simulink model "latest_exp"  (R2020a)
settings: Solver=ode1  StartTime=0.0  StopTime=20  FixedStep=0.001  RelTol=1e-3  EnableMultiTasking=on
PostLoadFcn:
  | qc_set_target_type(getConfigSet(bdroot, 'QUARC Default Target Configuration'));
model workspace (MAT data in the model file):
  b0 = 2500
values from neighbouring files (symbols this model uses):
  A = [0 0 1 0 ... (first row only)    [lqrintctrl.m]
  B = [0;0;51.5346;-49.3846]    [lqrintctrl.m]
  C = [1 0 0 0;0 1 0 0]    [lqrintctrl.m]
  D = [0;0]    [lqrintctrl.m]
libraries: simulink_extras x6, simulink x2
settings Model: ExtModeTrigDuration=10000  ExtModeTrigDurationFloating=10000  Creator=Rchan  LastModifiedBy=frank
settings SolverCC: PositivePriorityOrder=on
settings DataIOCC: LimitDataPoints=on  SaveFormat=Array  ReturnWorkspaceOutputs=off
settings OptimizationCC: ExpressionDepthLimit=2147483647  InitFltsAndDblsToZero=on  LifeSpan=inf
settings DebuggingCC: SaveWithParameterizedLinksMsg=none  UnderspecifiedInitializationDetection=Classic  MergeDetectMultiDrivingBlocksExec=none  SolverPrmCheckMsg=warning  MultiTaskDSMMsg=warning  MultiTaskCondExecSysMsg=none  FcnCallInpInsideContextMsg=warning  StateNameClashWarn=warning  SFUnexpectedBacktrackingDiag=warning  SFNoUnconditionalDefaultTransitionDiag=warning  SFExecutionAtInitializationDiag=none  ArithmeticOperatorsInVariantConditions=warning
settings HardwareCC: ProdBitPerPointer=32  ProdBitPerSizeT=32  ProdBitPerPtrDiffT=32  ProdLargestAtomicFloat=None  ProdIntDivRoundTo=Undefined  ProdEndianess=Unspecified  ProdWordSize=32  ProdHWDeviceType=32-bit Generic
settings ModelReferenceCC: PropagateSignalLabelsOutOfModel=off
settings SFSimCC: SimUseLocalCustomCode=off  CustomCodeUndefinedFunction=UseInterfaceOnly
settings RTWCC: Description=QUARC Win64 Target  SystemTargetFile=quarc_win64.tlc  TemplateMakefile=quarc_default_tmf  RTWUseLocalCustomCode=off
settings CodeAppCC: StateflowObjectComments=on
settings STFCustomTargetCC: TargetPreCompLibLocation=C:\PROGRA~3\QUARC\lib\2017a\win64\release  ConcurrentExecutionCompliant=on  CPPClassGenCompliant=on  GRTInterface=on  SystemTargetFile=quarc_win64.tlc
settings GRTTargetCC: TargetPreCompLibLocation=C:\PROGRA~3\QUARC\lib\2017a\win64\release  TargetLangStandard=C89/C90 (ANSI)  ParMdlRefBuildCompliant=off  CompOptLevelCompliant=off  CombineOutputUpdateFcns=off  MatFileLogging=off  GRTInterface=on  UseToolchainInfoCompliant=off  ExtMode=on  ExtModeMexFile=quarc_comm
settings ConfigComp: CovMetricSettings=dw  CovHtmlReporting=on  CovSaveCumulativeToWorkspaceVar=on  CovSaveSingleToWorkspaceVar=on  CovExternalEMLEnable=off

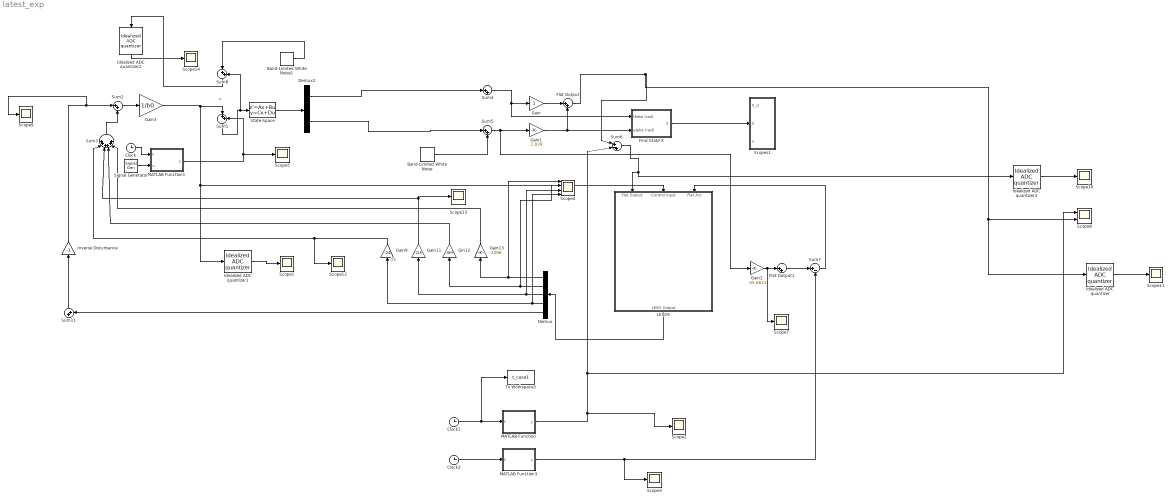
== system latest_exp ==
  note: -35
  note: u
  Band-Limited White Noise : simulink/Sources/Band-Limited White Noise  Cov=[1e-14]  Ts=0.001  seed=[2371]
  Band-Limited White Noise1 : simulink/Sources/Band-Limited White Noise  Cov=[1e-13]  Ts=0.001  seed=[2330]
  Clock : Clock
  Clock1 : Clock
  Clock2 : Clock
  Demux : Demux  Outputs=5
  Demux2 : Demux  Outputs=2
  Find State X : Subsystem
  Flat Output : Sum  Inputs=|++
  Flat Output1 : Sum  Inputs=|++
  Gain : Gain
  Gain1 : Gain  Gain=1.039
  Gain11 : Gain  Gain=-216
  Gain13 : Gain  Gain=-1296
  Gain2 : Gain  Gain=-45.6621
  Gain3 : Gain  Gain=1/b0
  Gain9 : Gain  Gain=-24
  Gin12 : Gain  Gain=-864
  Idealized ADC quantizer : simulink_extras/Additional Discrete/Idealized ADC quantizer  NumberOfConverterBits=12  Vmin=0  Vmax=5  OutputDataType=int16  OutputNegativeValues=off
  Idealized ADC quantizer1 : simulink_extras/Additional Discrete/Idealized ADC quantizer  NumberOfConverterBits=12  Vmin=-2  Vmax=2  OutputDataType=int16  OutputNegativeValues=on
  Idealized ADC quantizer2 : simulink_extras/Additional Discrete/Idealized ADC quantizer  NumberOfConverterBits=12  Vmin=-5  Vmax=5  OutputDataType=int16  OutputNegativeValues=on
  Idealized ADC quantizer3 : simulink_extras/Additional Discrete/Idealized ADC quantizer  NumberOfConverterBits=16  Vmin=-5  Vmax=5  OutputDataType=int16  OutputNegativeValues=on
  Inverse Disturbance : Gain  Gain=-1
  LESO5 : Subsystem
  MATLAB Function : MATLAB Function  TreatAsAtomicUnit=on
  MATLAB Function1 : MATLAB Function  TreatAsAtomicUnit=on
  MATLAB Function3 : MATLAB Function  TreatAsAtomicUnit=on
  Scope{1..3,5,7,9..14} (11 alike) : Scope
  Scope4 : Scope  NumInputPorts=4
  Scope8 : Scope  NumInputPorts=2
  Scopes1 : Subsystem
  Signal Generator : SignalGenerator  WaveForm=square  Amplitude=0.05  Frequency=0.5  Units=rad/sec
  State-Space : StateSpace  A=A  B=B  C=C  D=D  InitialCondition=[0,0,0,0]
  Sum{1..2,4..5,8,11} (6 alike) : Sum  Inputs=|++
  Sum3 : Sum  Inputs=++++++
  Sum6 : Sum  Inputs=|+-+
  Sum7 : Sum  Inputs=|+-
  To Workspace3 : ToWorkspace  VariableName=t_case1  SampleTime=-1
  wires:
  MATLAB Function3/1(y) -> Scope3/1, Sum7/2
  Clock2/1 -> MATLAB Function3/1(t)
  Gain13/1 -> Sum3/5
  Demux/3 -> Scope4/3, Gain11/1
  Sum2/1 -> Gain3/1
  Demux/5 -> Sum11/2
  Find State X/1(X) -> Scopes1/2(X)
  Demux/4 -> Gain9/1, Scope4/4
  Gain2/1 -> Scope7/1, Flat Output1/1
  Sum3/1 -> Sum2/2
  Sum11/1 -> Inverse Disturbance/1
  Gain9/1 -> Scope12/1, Sum3/2
  Gain3/1 -> Sum1/1, Idealized ADC quantizer1/1, LESO5/2(Control Input)
  Sum6/1 -> Idealized ADC quantizer3/1, LESO5/1(Flat Output)
  Flat Output1/1 -> Sum7/1
  MATLAB Function/1(y) -> Scope2/1, Sum6/2, Scope8/1
  Inverse Disturbance/1 -> Scope9/1, Sum2/1
  Sum4/1 -> Find State X/1(theta (rad)), Gain/1
  Sum7/1 -> LESO5/3("Flat Acc ")
  Gain11/1 -> Scope13/1, Sum3/3
  Demux/2 -> Scope4/2, Gin12/1
  Demux/1 -> Scope4/1, Gain13/1
  Demux2/1 -> Sum4/1
  Demux2/2 -> Sum5/1
  Gin12/1 -> Sum3/4
  LESO5/1(LESO Output) -> Demux/1
  Gain1/1 -> Find State X/2(alpha (rad)), Flat Output/2
  Gain/1 -> Flat Output/1
  Sum5/1 -> Gain2/1, Gain1/1
  Clock1/1 -> To Workspace3/1, MATLAB Function/1(t)
  State-Space/1 -> Demux2/1
  Idealized ADC quantizer/1 -> Scope11/1
  Idealized ADC quantizer1/1 -> Scope1/1
  Signal Generator/1 -> MATLAB Function1/2(u)
  MATLAB Function1/1(y) -> Scope5/1, Sum1/2
  Sum1/1 -> Sum8/2, State-Space/1
  Clock/1 -> MATLAB Function1/1(t)
  Band-Limited White Noise1/1 -> Sum8/1
  Flat Output/1 -> Idealized ADC quantizer/1, Scope8/2, Sum6/1
  Band-Limited White Noise/1 -> Sum5/2
  Sum8/1 -> Idealized ADC quantizer2/1
  Idealized ADC quantizer2/1 -> Scope14/1
  Idealized ADC quantizer3/1 -> Scope10/1

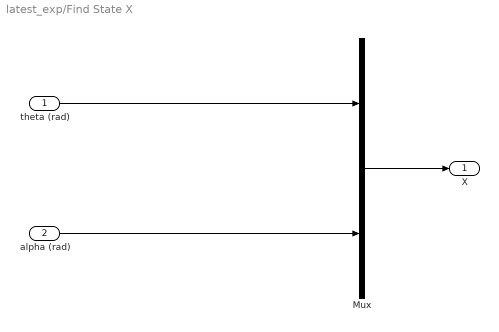
== system latest_exp/Find State X ==
  theta (rad) : Inport
  alpha (rad) : Inport  Port=2
  Mux : Mux  Inputs=2
  X : Outport
  wires:
  alpha (rad)/1 -> Mux/2
  Mux/1 -> X/1
  theta (rad)/1 -> Mux/1

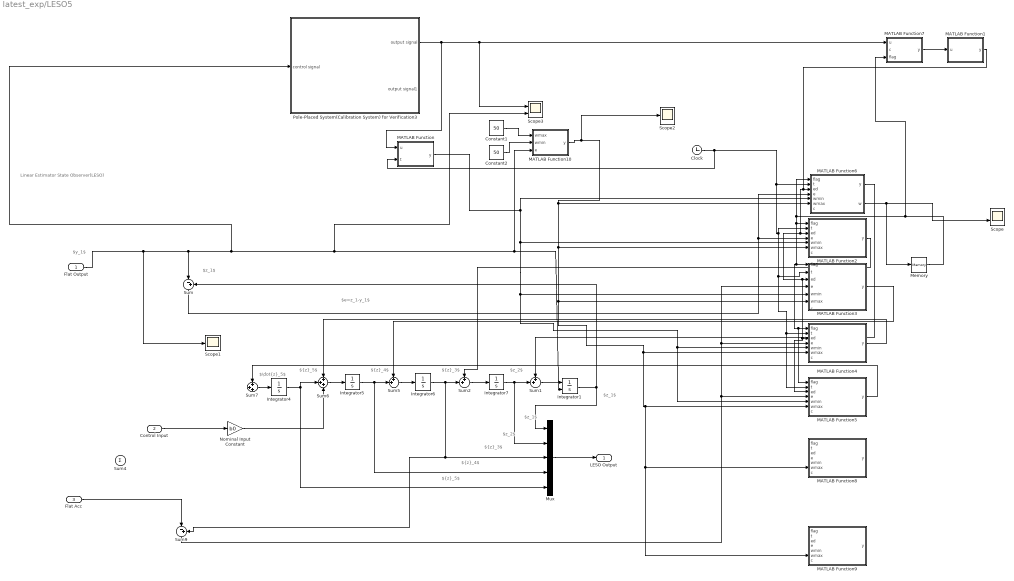
== system latest_exp/LESO5 ==
  note: $e=z_1-y_1$
  note: ${z}_5$
  note: $\dot{z}_5$
  note: ${z}_4$
  note: ${z}_3$
  note: $z_2$
  note: $z_1$
  note: $y_1$
  note: $z_1$
  note: Linear Estimator State Observer(LESO)
  note: $z_1$
  note: $z_2$
  note: ${z}_3$
  note: ${z}_4$
  note: ${z}_5$
  Flat Output : Inport
  Control Input : Inport  Port=2
  "Flat Acc " : Inport  Port=3
  Clock : Clock
  Constant1 : Constant  Value=50
  Constant2 : Constant  Value=50
  Integrator1 : Integrator  InitialConditionSource=external
  Integrator{4..7} (4 alike) : Integrator
  MATLAB Function : MATLAB Function  TreatAsAtomicUnit=on
  MATLAB Function1 : MATLAB Function  TreatAsAtomicUnit=on
  MATLAB Function10 : MATLAB Function  TreatAsAtomicUnit=on
  MATLAB Function2 : MATLAB Function  TreatAsAtomicUnit=on
  MATLAB Function3 : MATLAB Function  TreatAsAtomicUnit=on
  MATLAB Function4 : MATLAB Function  TreatAsAtomicUnit=on
  MATLAB Function5 : MATLAB Function  TreatAsAtomicUnit=on
  MATLAB Function6 : MATLAB Function  TreatAsAtomicUnit=on
  MATLAB Function7 : MATLAB Function  TreatAsAtomicUnit=on
  MATLAB Function8 : MATLAB Function  TreatAsAtomicUnit=on
  MATLAB Function9 : MATLAB Function  TreatAsAtomicUnit=on
  Memory : Memory
  Mux : Mux  Inputs=5
  Nominal Input Constant : Gain  Gain=b0
  Pole-Placed System(Calibration System) for Verification3 : Subsystem
  Scope : Scope  NumInputPorts=2
  Scope1 : Scope
  Scope2 : Scope
  Scope3 : Scope  NumInputPorts=2
  Sum : Sum  Inputs=|-+
  Sum1 : Sum  Inputs=++|
  Sum2 : Sum  Inputs=++|
  Sum4 : Sum  Inputs=+|
  Sum5 : Sum  Inputs=++|
  Sum6 : Sum  Inputs=+++
  Sum7 : Sum  Inputs=+++
  Sum9 : Sum  Inputs=|-+
  LESO Output : Outport
  wires:
  Integrator7/1 -> Mux/2, Sum1/2
  Integrator6/1 -> Sum9/2, Mux/3, Sum2/2
  Sum1/1 -> Integrator1/1
  Integrator4/1 -> Mux/5, Sum6/2
  Nominal Input Constant/1 -> Sum6/3
  Mux/1 -> LESO Output/1
  Sum2/1 -> Integrator7/1
  Sum5/1 -> Integrator6/1
  Integrator1/1 -> Sum/2, Mux/1
  Control Input/1 -> Nominal Input Constant/1
  Sum6/1 -> Integrator5/1
  Sum7/1 -> Integrator4/1
  Integrator5/1 -> Mux/4, Sum5/2
  MATLAB Function10/1(y) -> Scope2/1, MATLAB Function9/6(wmax), MATLAB Function8/6(wmax), MATLAB Function5/6(wmax), MATLAB Function4/6(wmax), MATLAB Function3/6(wmax), MATLAB Function2/6(wmax), MATLAB Function6/6(wmax)
  MATLAB Function/1(y) -> MATLAB Function5/5(wmin), MATLAB Function4/5(wmin), MATLAB Function3/5(wmin), MATLAB Function2/5(wmin), MATLAB Function6/5(wmin)
  ? -> MATLAB Function7/2(c), MATLAB Function5/7(c), MATLAB Function4/7(c), MATLAB Function3/7(c), MATLAB Function2/7(c), MATLAB Function6/7(c)
  MATLAB Function6/1(y) -> Sum1/1
  MATLAB Function2/1(y) -> Sum2/1
  MATLAB Function4/1(y) -> Sum6/1
  MATLAB Function5/1(y) -> Sum7/1
  Clock/1 -> MATLAB Function/2(t), MATLAB Function4/2(t), MATLAB Function5/2(t), MATLAB Function3/2(t), MATLAB Function2/2(t), MATLAB Function6/2(t)
  MATLAB Function6/2(w) -> Memory/1, Scope/2
  Flat Output/1 -> Scope1/1, Pole-Placed System(Calibration System) for Verification3/1(control signal), MATLAB Function10/3(e), Integrator1/2, Scope3/2, Sum/1
  Pole-Placed System(Calibration System) for Verification3/1(output signal) -> MATLAB Function/1(u), Scope3/1, MATLAB Function7/1(u)
  Memory/1 -> MATLAB Function7/3(flag), MATLAB Function2/1(flag), MATLAB Function3/1(flag), MATLAB Function4/1(flag), MATLAB Function5/1(flag), MATLAB Function6/1(flag)
  MATLAB Function7/1(y) -> MATLAB Function1/1(u)
  MATLAB Function1/1(y) -> MATLAB Function5/3(ed), MATLAB Function4/3(ed), MATLAB Function3/3(ed), MATLAB Function2/3(ed), MATLAB Function6/3(ed)
  Sum/1 -> MATLAB Function2/4(e), MATLAB Function6/4(e)
  MATLAB Function3/1(y) -> Sum5/1
  "Flat Acc "/1 -> Sum9/1
  Sum9/1 -> MATLAB Function3/4(e), MATLAB Function4/4(e), MATLAB Function5/4(e)
  Constant1/1 -> MATLAB Function10/1(wmax)
  Constant2/1 -> MATLAB Function10/2(wmin)

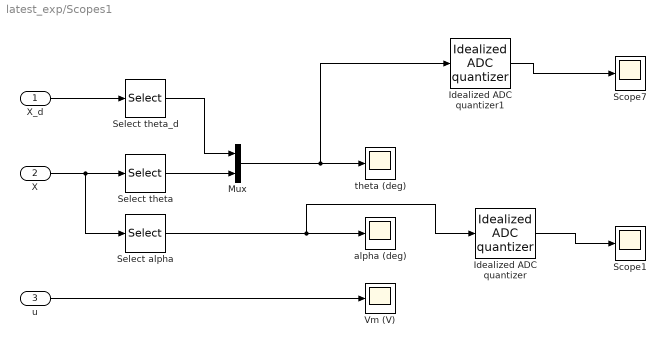
== system latest_exp/Scopes1 ==
  X_d : Inport
  X : Inport  Port=2
  u : Inport  Port=3
  Idealized ADC quantizer : simulink_extras/Additional Discrete/Idealized ADC quantizer  NumberOfConverterBits=12  Vmin=-2  Vmax=2  OutputDataType=int16  OutputNegativeValues=on
  Idealized ADC quantizer1 : simulink_extras/Additional Discrete/Idealized ADC quantizer  NumberOfConverterBits=12  Vmin=0  Vmax=5  OutputDataType=single  OutputNegativeValues=off
  Mux : Mux  Inputs=2
  Scope1 : Scope
  Scope7 : Scope
  Select alpha : Selector  InputPortWidth=2  IndexOptions=Index vector (dialog)  Indices=2  OutputSizes=[(-2)]
  Select theta : Selector  InputPortWidth=2  IndexOptions=Index vector (dialog)  Indices=1  OutputSizes=[(-2)]
  Select theta_d : Selector  InputPortWidth=4  IndexOptions=Index vector (dialog)  Indices=1  OutputSizes=[(-2)]
  Vm (V) : Scope
  alpha (deg) : Scope
  theta (deg) : Scope
  wires:
  u/1 -> Vm (V)/1
  X_d/1 -> Select theta_d/1
  X/1 -> Select alpha/1, Select theta/1
  Select theta_d/1 -> Mux/1
  Select theta/1 -> Mux/2
  Select alpha/1 -> Idealized ADC quantizer/1, alpha (deg)/1
  Mux/1 -> Idealized ADC quantizer1/1, theta (deg)/1
  Idealized ADC quantizer/1 -> Scope1/1
  Idealized ADC quantizer1/1 -> Scope7/1

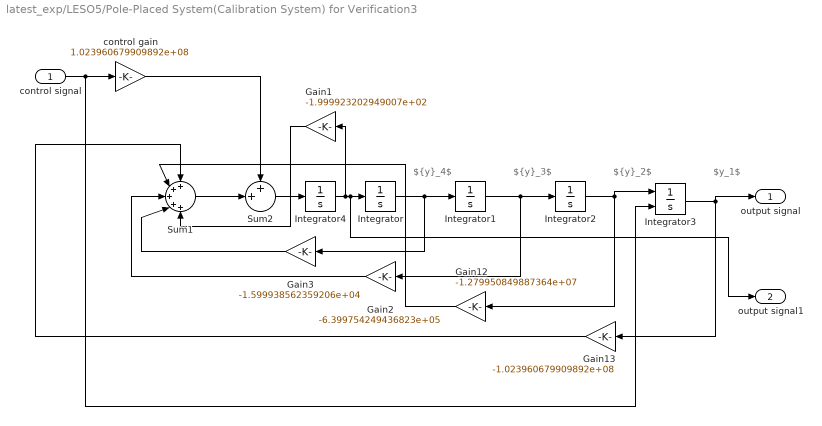
== system latest_exp/LESO5/Pole-Placed System(Calibration System) for Verification3 ==
  note: ${y}_4$
  note: ${y}_3$
  note: ${y}_2$
  note: $y_1$
  control signal : Inport
  Gain1 : Gain  Gain=-1.999923202949007e+02
  Gain12 : Gain  Gain=-1.279950849887364e+07
  Gain13 : Gain  Gain=-1.023960679909892e+08
  Gain2 : Gain  Gain=-6.399754249436823e+05
  Gain3 : Gain  Gain=-1.599938562359206e+04
  Integrator{,1..2,4} (4 alike) : Integrator
  Integrator3 : Integrator  InitialConditionSource=external
  Sum1 : Sum  Inputs=+++++
  Sum2 : Sum  Inputs=++|
  control gain : Gain  Gain=1.023960679909892e+08
  output signal : Outport
  output signal1 : Outport  Port=2
  wires:
  Integrator2/1 -> Gain12/1, Integrator3/1
  Gain3/1 -> Sum1/4
  Integrator/1 -> Gain3/1, Integrator1/1
  Gain12/1 -> Sum1/2
  Integrator3/1 -> output signal/1, Gain13/1
  Integrator1/1 -> Gain2/1, Integrator2/1
  Gain2/1 -> Sum1/3
  Gain13/1 -> Sum1/1
  Sum1/1 -> Sum2/2
  Sum2/1 -> Integrator4/1
  control gain/1 -> Sum2/1
  Integrator4/1 -> Gain1/1, output signal1/1, Integrator/1
  Gain1/1 -> Sum1/5
  control signal/1 -> Integrator3/2, control gain/1

== matlab function latest_exp/LESO5/MATLAB Function5 ==
  data: flag input; t input; ed input; e input; y output; wmin input; wmax input; c input
function y = fcn(flag,t,ed,e,wmin,wmax,c)
% if t<5.5
% w=wmax-(wmax-wmin)*tanh(c*t);
% else
% w=wmin+(wmax-wmin)*tanh(c*(t-5.5));
% end 

% w=wmin+(wmax-wmin)*tanh(c*abs(ed)^2);
% w=wmin+(wmax-wmin)*ed;
w=wmax;
y = -w^3*e;  
end

== matlab function latest_exp/LESO5/MATLAB Function6 ==
  data: flag input; t input; ed input; e input; y output; wmin input; wmax input; c input; w output
function [y,w] = fcn(flag,t,ed,e,wmin,wmax,c)
% if abs(t) < 0.1
%     %w=wmin+(wmax-wmin)*tanh(c*abs(t));
%     w=wmax;
% else

%w=wmin+(wmax-wmin)*tanh(c*tanh(0.0025*flag)*abs(ed)^2);
%w=wmin+(wmax-wmin)*tanh(c*abs(ed)^2);
%=wmin+(wmax-wmin)*tanh(c*t);
w=wmax;
%w=wmin+(wmax-wmin)*ed+50;
    
% w=wmin+(wmax-wmin)*tanh(c*abs(e));
y = -2*w*e;               
end

== matlab function latest_exp/MATLAB Function ==
  data: t input; y output
function y = fcn(t)
if t<2
    y=0;
elseif (t>=2 && t<=6)
y=1*(-5/4096*(t-2)^7 + 35/2048*(t-2)^6 - 21/256*(t-2)^5 + 35/256*(t-2)^4);
else
   y=1
end

== matlab function latest_exp/MATLAB Function3 ==
  data: t input; y output
function y = fcn(t)
if t<2
    y=0;
elseif (t>=2 && t<=6)
y=1*(-5/4096*7*6*(t-2).^5 + 35/2048*6*5*(t-2).^4 - 21/256*5*4*(t-2).^3 + 35/256*4*3*(t-2).^2);
else
   y=0
end

== matlab function latest_exp/LESO5/MATLAB Function ==
  data: u input; y output; t input
function y = fcn(u,t)
% if u <0.5
%y = 100-(100-75)*tanh(0.01*t);
% else
y=100;
end

== matlab function latest_exp/LESO5/MATLAB Function1 ==
  data: u input; y output
function y = fcn(u)
if u<=0.05
    y=u
else
    y=tanh(u)
    
end

== matlab function latest_exp/LESO5/MATLAB Function7 ==
  data: u input; y output; c input; flag input
function y = fcn(u,c,flag)
y = c*abs(u);

== matlab function latest_exp/LESO5/MATLAB Function2 ==
  data: flag input; t input; ed input; e input; y output; wmin input; wmax input; c input
function y = fcn(flag,t,ed,e,wmin,wmax,c)

% if t<5.5
% w=wmax-(wmax-wmin)*tanh(c*t);
% else
% w=wmin+(wmax-wmin)*tanh(c*(t-5.5));
% end 

% w=wmin+(wmax-wmin)*tanh(c*abs(ed)^2);
% w=wmin+(wmax-wmin)*ed;
w=wmax;
% w=wmin+(wmax-wmin)*tanh(c*abs(e));
y = -w^2*e;               
end

== matlab function latest_exp/LESO5/MATLAB Function8 ==
  data: flag input; t input; ed input; e input; y output; wmin input; wmax input; c input
function y = fcn(flag,t,ed,e,wmin,wmax,c)
% if t<5.5
% w=wmax-(wmax-wmin)*tanh(c*t);
% else
% w=wmin+(wmax-wmin)*tanh(c*(t-5.5));
% end 

% w=wmin+(wmax-wmin)*tanh(c*abs(ed)^2);
% w=wmin+(wmax-wmin)*ed;
w=wmax;
y = -5*w^4*e;               
end

== matlab function latest_exp/LESO5/MATLAB Function9 ==
  data: flag input; t input; ed input; e input; y output; wmin input; wmax input; c input
function y = fcn(flag,t,ed,e,wmin,wmax,c)
% if t<5.5
% w=wmax-(wmax-wmin)*tanh(c*t);
% else
% w=wmin+(wmax-wmin)*tanh(c*(t-5.5));
% end 

% w=wmin+(wmax-wmin)*tanh(c*abs(ed)^2);
% w=wmin+(wmax-wmin)*ed;
w=wmax;
y = -w^5*e;               
end

== matlab function latest_exp/LESO5/MATLAB Function10 ==
  data: wmax input; wmin input; y output; e input
function y = fcn(wmax,wmin,e)
%y=wmin+(wmax-wmin)*tanh(20*abs(e));;
y=wmax;
end

== matlab function latest_exp/MATLAB Function1 ==
  data: t input; u input; y output
function y = fcn(t, u)
if t<12 && t>11
    y=u;
else
    y=0;
end

== matlab function latest_exp/LESO5/MATLAB Function3 ==
  data: flag input; t input; ed input; e input; y output; wmin input; wmax input; c input
function y = fcn(flag,t,ed,e,wmin,wmax,c)

% if t<5.5
% w=wmax-(wmax-wmin)*tanh(c*t);
% else
% w=wmin+(wmax-wmin)*tanh(c*(t-5.5));
% end 

%w=wmin+(wmax-wmin)*tanh(c*abs(ed)^2);
% w=wmin+(wmax-wmin)*ed;
w=wmax;
y = -3*w*e; 
end

== matlab function latest_exp/LESO5/MATLAB Function4 ==
  data: flag input; t input; ed input; e input; y output; wmin input; wmax input; c input
function y = fcn(flag,t,ed,e,wmin,wmax,c)
% if t<5.5
% w=wmax-(wmax-wmin)*tanh(c*t);
% else
% w=wmin+(wmax-wmin)*tanh(c*(t-5.5));
% end 

% w=wmin+(wmax-wmin)*tanh(c*abs(ed)^2);
% w=wmin+(wmax-wmin)*ed;
w=wmax;
y = -3*w^2*e;   
end
